simulink model "lab03z3b_sch"  (R2021a)
settings: Solver=VariableStepAuto  StartTime=0.0  StopTime=80  MaxStep=0.001  RelTol=1e-3
values from neighbouring files (symbols this model uses):
  fw = 1/40    (= 0.025)    [lab03z3.m]
  K = -place(A, B, s)    [lab03z3.m]
settings Model: Creator=user  LastModifiedBy=AgraWoodAdmin
settings SolverCC: AlgebraicLoopSolver=TrustRegion
settings DataIOCC: ReturnWorkspaceOutputs=off
settings DebuggingCC: SFMachineParentedDataDiag=warning  ArithmeticOperatorsInVariantConditions=warning
settings SFSimCC: SimUseLocalCustomCode=off  CustomCodeUndefinedFunction=UseInterfaceOnly
settings RTWCC: RTWUseLocalCustomCode=off

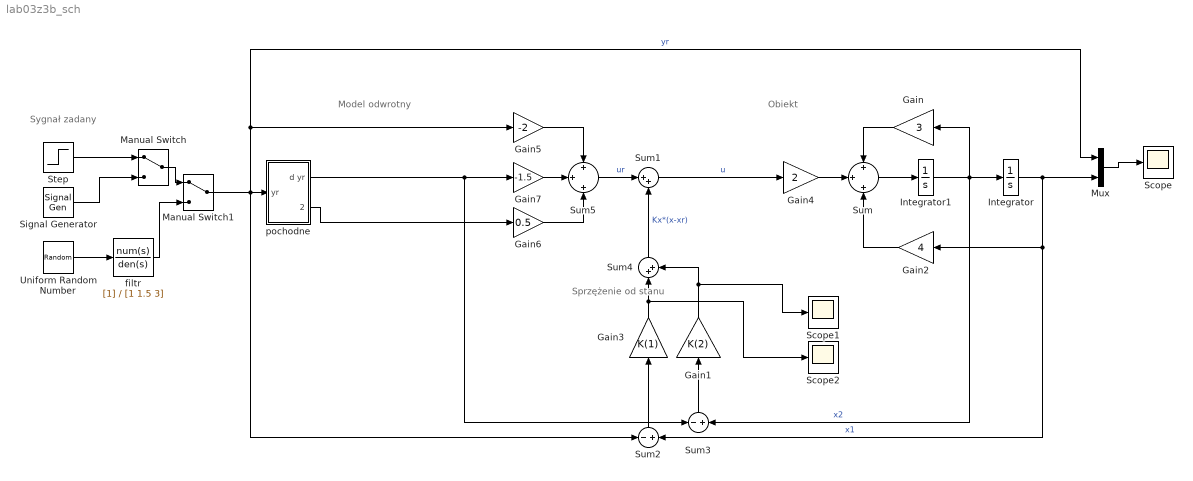
== system lab03z3b_sch ==
  note: Sygnał zadany
  note: Model
      | odwrotny
  note: Sprzężenie
      | od stanu
  note: Obiekt
  Gain : Gain  Gain=3
  Gain1 : Gain  Gain=K(2)
  Gain2 : Gain  Gain=4
  Gain3 : Gain  Gain=K(1)
  Gain4 : Gain  Gain=2
  Gain5 : Gain  Gain=-2
  Gain6 : Gain  Gain=0.5
  Gain7 : Gain  Gain=-1.5
  Integrator : Integrator
  Integrator1 : Integrator
  Manual Switch : ManualSwitch
  Manual Switch1 : ManualSwitch
  Mux : Mux  Inputs=2
  Scope : Scope
  Scope1 : Scope
  Scope2 : Scope
  Signal Generator : SignalGenerator  Amplitude=2  Frequency=fw
  Step : Step  SampleTime=0
  Sum : Sum  Inputs=+|+|+
  Sum1 : Sum  Inputs=|++
  Sum2 : Sum  Inputs=-|+
  Sum3 : Sum  Inputs=-|+
  Sum4 : Sum  Inputs=|++
  Sum5 : Sum  Inputs=+|+|+
  Uniform Random Number : UniformRandomNumber  Minimum=-0.5  Maximum=0.5  Seed=100  SampleTime=5
  filtr : TransferFcn  Denominator=[1 1.5 3]
  pochodne : Subsystem
  wires:
  Sum/1 -> Integrator1/1
  Gain/1 -> Sum/1
  Gain2/1 -> Sum/3
  Gain4/1 -> Sum/2
  Sum4/1 -> Sum1/2  "Kx*(x-xr)"
  Integrator1/1 -> Sum3/2, Integrator/1, Gain/1  "x2"
  Integrator/1 -> Mux/2, Sum2/2, Gain2/1  "x1"
  Sum2/1 -> Gain3/1
  Sum3/1 -> Gain1/1
  Gain3/1 -> Sum4/1, Scope2/1
  Gain1/1 -> Scope1/1, Sum4/2
  pochodne/1(d yr) -> Sum3/1, Gain7/1
  Gain6/1 -> Sum5/3
  Gain7/1 -> Sum5/2
  Gain5/1 -> Sum5/1
  Sum5/1 -> Sum1/1  "ur"
  Sum1/1 -> Gain4/1  "u"
  Step/1 -> Manual Switch/1
  Manual Switch1/1 -> Gain5/1, Mux/1, pochodne/1(yr), Sum2/1  "yr"
  Signal Generator/1 -> Manual Switch/2
  Mux/1 -> Scope/1
  Uniform Random Number/1 -> filtr/1
  Manual Switch/1 -> Manual Switch1/1
  filtr/1 -> Manual Switch1/2
  pochodne/2(dd yr) -> Gain6/1

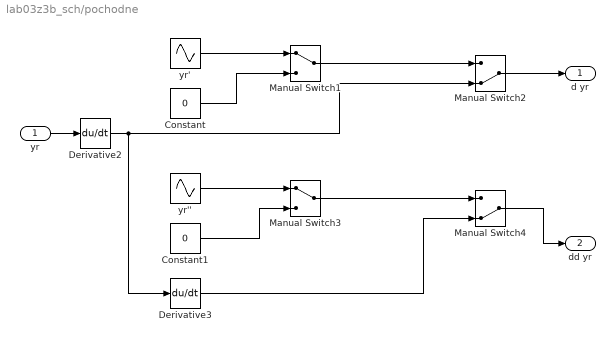
== system lab03z3b_sch/pochodne ==
  yr : Inport
  Constant : Constant  Value=0
  Constant1 : Constant  Value=0
  Derivative2 : Derivative
  Derivative3 : Derivative
  Manual Switch1 : ManualSwitch
  Manual Switch2 : ManualSwitch  CurrentSetting=0
  Manual Switch3 : ManualSwitch
  Manual Switch4 : ManualSwitch  CurrentSetting=0
  yr' : Sin  Amplitude=2*(2*pi*fw)  Frequency=2*pi*fw  Phase=pi/2  SampleTime=0
  yr'' : Sin  Amplitude=-2*(2*pi*fw)^2  Frequency=2*pi*fw  SampleTime=0
  d yr : Outport  VectorParamsAs1DForOutWhenUnconnected=off
  dd yr : Outport  Port=2  VectorParamsAs1DForOutWhenUnconnected=off
  wires:
  yr/1 -> Derivative2/1
  Constant/1 -> Manual Switch1/2
  Constant1/1 -> Manual Switch3/2
  Manual Switch4/1 -> dd yr/1
  yr'/1 -> Manual Switch1/1
  Derivative2/1 -> Manual Switch2/2, Derivative3/1
  yr''/1 -> Manual Switch3/1
  Manual Switch3/1 -> Manual Switch4/1
  Derivative3/1 -> Manual Switch4/2
  Manual Switch2/1 -> d yr/1
  Manual Switch1/1 -> Manual Switch2/1
